simulink model "Invertedpendulumsim"  (R2023a)
settings: Solver=VariableStepAuto  StartTime=0.0  StopTime=10.0  MaxStep=0.01  MinStep=0.0001  RelTol=1e-6
values from neighbouring files (symbols this model uses):
  A = [0 1 0 0;8.175 0 0 0; 0 0 0 1; -3.27 0 0 0]    [inverted_pend_script.m]
  B = [0;-0.33; 0; 0.467]    [inverted_pend_script.m]
  K = acker(A_bar,B_bar,[-4+2i -4-2i -10 -10 -10])    [inverted_pend_script.m]
settings Model: Creator=siddi  LastModifiedBy=bikra
settings DebuggingCC: UnconnectedInputMsg=warning  UnconnectedOutputMsg=warning  UnconnectedLineMsg=warning
settings ModelReferenceCC: EnableRefExpFcnMdlSchedulingChecks=on
settings RTWCC: DLArmComputeVersion=19.05

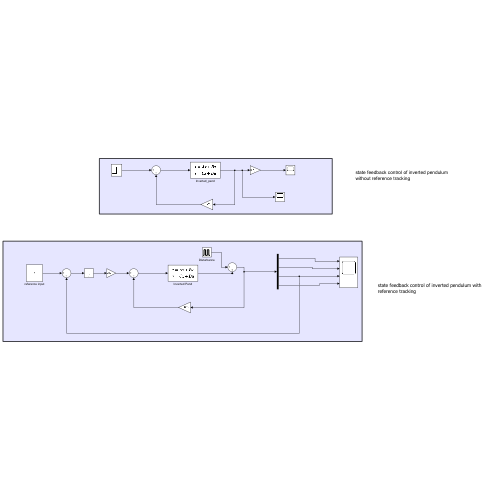
[thumbnail: Simulink's stored preview of the top-level diagram]
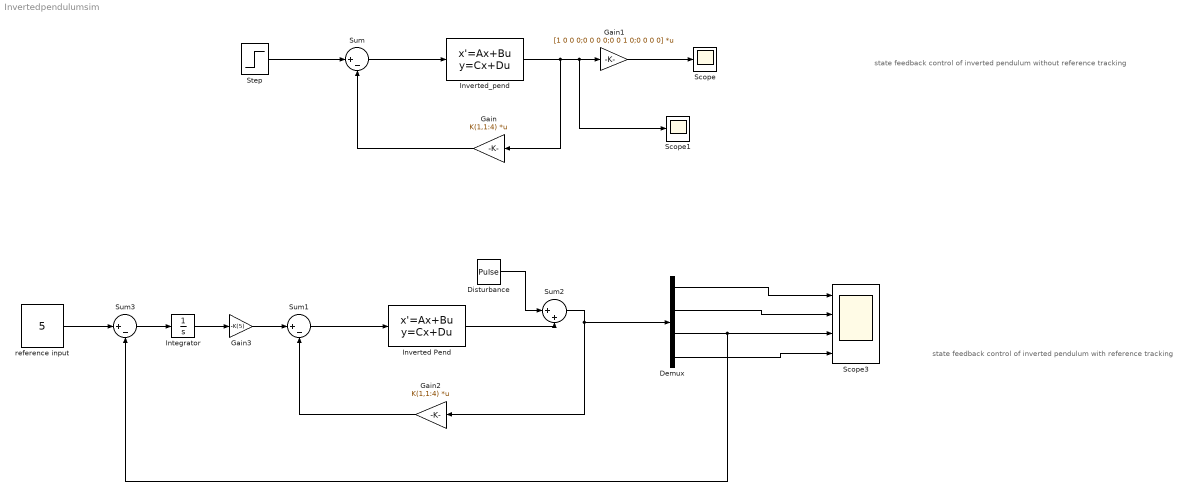
== system Invertedpendulumsim ==
  note: state feedback control of inverted pendulum with reference tracking
  note: state feedback control of inverted pendulum without reference tracking
  Demux : Demux
  Disturbance : DiscretePulseGenerator  PulseType=Time based  Period=10  PulseWidth=5
  Gain : Gain  Gain=K(1,1:4)  Multiplication=Matrix(K*u)
  Gain1 : Gain  Gain=[1 0 0 0;0 0 0 0;0 0 1 0;0 0 0 0]  Multiplication=Matrix(K*u)
  Gain2 : Gain  Gain=K(1,1:4)  Multiplication=Matrix(K*u)
  Gain3 : Gain  Gain=-K(5)
  Integrator : Integrator
  Inverted Pend : StateSpace  A=A  B=B  C=eye(4)  D=zeros(4,1)  InitialCondition=[2 2 0 0];
  Inverted_pend : StateSpace  A=A  B=B  C=eye(4)  D=zeros(4,1)  InitialCondition=[2 2 0 0];
  Scope : Scope
  Scope1 : Scope
  Scope3 : Scope  NumInputPorts=4
  Step : Step  SampleTime=0
  Sum : Sum  Inputs=|+-
  Sum1 : Sum  Inputs=|+-
  Sum2 : Sum  Inputs=|++
  Sum3 : Sum  Inputs=|+-
  reference input : Constant  Value=5
  wires:
  Step/1 -> Sum/1
  Sum/1 -> Inverted_pend/1
  Inverted_pend/1 -> Gain/1, Scope1/1, Gain1/1
  Gain1/1 -> Scope/1
  Gain/1 -> Sum/2
  Gain2/1 -> Sum1/2
  Sum1/1 -> Inverted Pend/1
  Inverted Pend/1 -> Sum2/2
  Sum2/1 -> Demux/1, Gain2/1
  Disturbance/1 -> Sum2/1
  Demux/1 -> Scope3/1
  Demux/2 -> Scope3/2
  Demux/3 -> Sum3/2, Scope3/3
  Demux/4 -> Scope3/4
  Gain3/1 -> Sum1/1
  Integrator/1 -> Gain3/1
  Sum3/1 -> Integrator/1
  reference input/1 -> Sum3/1
